simulink model "Simu_SpeedEstimation"  (R2018b)
settings: Solver=FixedStepAuto  StartTime=0.0  StopTime=60  FixedStep=.00005  RelTol=1e-3
undefined symbols (not defined in the file or in its folder): DiscIntNeverNeededParam, sim2mat
libraries: dsparch4 x1, simulink x1
settings Model: Creator=Lubin Kerhuel  LastModifiedBy=Lubin Kerhuel

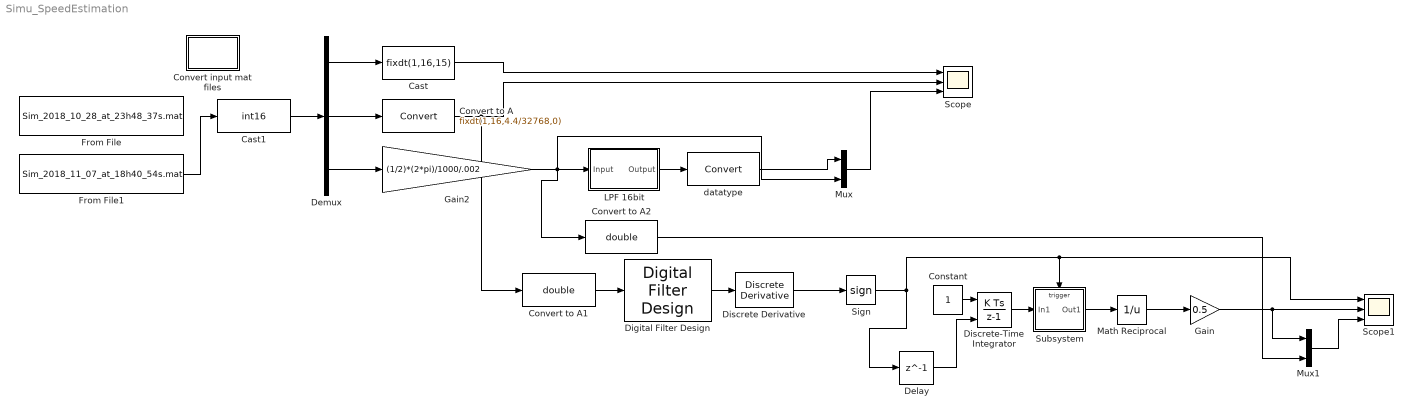
== system Simu_SpeedEstimation ==
  Cast : DataTypeConversion  OutDataTypeStr=fixdt(1,16,15)  ConvertRealWorld=Stored Integer (SI)
  Cast1 : DataTypeConversion  OutDataTypeStr=int16
  Constant : Constant
  Convert input mat files : Subsystem  LoadFcn=sim2mat();
      settings: OpenFcn=sim2mat();
  Convert to A : DataTypeConversion  OutDataTypeStr=fixdt(1,16,4.4/32768,0)  ConvertRealWorld=Stored Integer (SI)
  Convert to A1 : DataTypeConversion  OutDataTypeStr=double
  Convert to A2 : DataTypeConversion  OutDataTypeStr=double
  Delay : Delay  DelayLength=1  InitialCondition=0
  Demux : Demux  Outputs=3
  Digital Filter Design : dsparch4/Digital Filter Design  mwdsp_browser_bugfix_var=off
  Discrete Derivative : simulink/Discrete/Discrete Derivative  gainval=1  ICPrevScaledInput=0  OutMin=[]  OutMax=[]  OutDataType=fixdt(1, 16)  OutScaling=2^-10  DoSatur=off
  Discrete-Time Integrator : DiscreteIntegrator  ExternalReset=rising  SampleTime=-1  ICPrevOutput=DiscIntNeverNeededParam  ICPrevScaledInput=DiscIntNeverNeededParam
  From File : FromFile  FileName=Sim_2018_10_28_at_23h48_37s.mat  SampleTime=.00005
  From File1 : FromFile  FileName=Sim_2018_11_07_at_18h40_54s.mat  SampleTime=.00005
  Gain : Gain  Gain=0.5
  Gain2 : Gain  Gain=(1/2)*(2*pi)/1000/.002  OutDataTypeStr=fixdt(1,16,5)  LockScale=on
  "LPF 16bit " : Subsystem  Tag=FilterWizardSubSystem
      settings: ErrorFcn=dspFilterRealizedInBasicElemsAlgLoopErrFcnCallback
  Math Reciprocal : Math  Operator=reciprocal  SaturateOnIntegerOverflow=on
  Mux : Mux  Inputs=2
  Mux1 : Mux  Inputs=2
  Scope : Scope  NumInputPorts=3
  Scope1 : Scope  NumInputPorts=3
  Sign : Signum
  Subsystem : Subsystem
  datatype : DataTypeConversion
  wires:
  From File1/1 -> Cast1/1
  Demux/1 -> Cast/1
  Demux/2 -> Convert to A/1
  Demux/3 -> Gain2/1
  Cast/1 -> Scope/1
  Convert to A/1 -> Convert to A1/1, Scope/2
  Gain2/1 -> Convert to A2/1, Mux/2, "LPF 16bit "/1(Input)
  Cast1/1 -> Demux/1
  "LPF 16bit "/1(Output) -> datatype/1
  Mux/1 -> Scope/3
  datatype/1 -> Mux/1
  Discrete-Time Integrator/1 -> Subsystem/1(In1)
  Discrete Derivative/1 -> Sign/1
  Constant/1 -> Discrete-Time Integrator/1
  Digital Filter Design/1 -> Discrete Derivative/1
  Convert to A1/1 -> Digital Filter Design/1
  Subsystem/1(Out1) -> Math Reciprocal/1
  Sign/1 -> Delay/1, Subsystem/Trigger, Scope1/1
  Delay/1 -> Discrete-Time Integrator/2
  Math Reciprocal/1 -> Gain/1
  Gain/1 -> Mux1/1, Scope1/2
  Mux1/1 -> Scope1/3
  Convert to A2/1 -> Mux1/2

== system Simu_SpeedEstimation/Convert input mat files ==

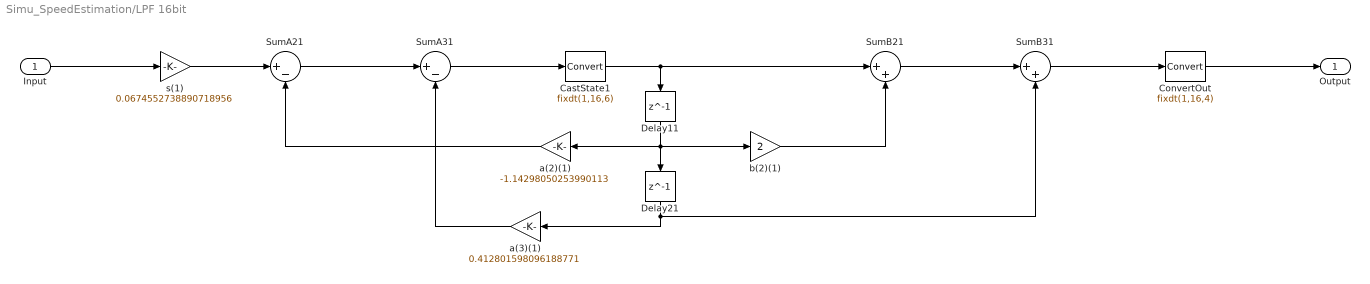
== system Simu_SpeedEstimation/LPF 16bit  ==
  Input : Inport
  CastState1 : DataTypeConversion  OutDataTypeStr=fixdt(1,16,6)
  ConvertOut : DataTypeConversion  OutDataTypeStr=fixdt(1,16,4)
  Delay11 : Delay  DelayLength=1  InitialCondition=0
  Delay21 : Delay  DelayLength=1  InitialCondition=0
  SumA21 : Sum  Inputs=|+-  AccumDataTypeStr=fixdt(1,16,6)  OutDataTypeStr=fixdt(1,16,6)
  SumA31 : Sum  Inputs=|+-  AccumDataTypeStr=fixdt(1,16,6)  OutDataTypeStr=fixdt(1,16,6)
  SumB21 : Sum  Inputs=|++  AccumDataTypeStr=fixdt(1,16,5)  OutDataTypeStr=fixdt(1,16,5)
  SumB31 : Sum  Inputs=|++  AccumDataTypeStr=fixdt(1,16,4)  OutDataTypeStr=fixdt(1,16,4)
  a(2)(1) : Gain  Gain=-1.14298050253990113  ParamDataTypeStr=fixdt(1,16,14)  OutDataTypeStr=fixdt(1,16,6)
  a(3)(1) : Gain  Gain=0.412801598096188771  ParamDataTypeStr=fixdt(0,16,17)  OutDataTypeStr=fixdt(1,16,8)
  b(2)(1) : Gain  Gain=2  ParamDataTypeStr=fixdt(0,16,14)  OutDataTypeStr=fixdt(1,16,5)
  s(1) : Gain  Gain=0.0674552738890718956  ParamDataTypeStr=fixdt(0,16,19)  OutDataTypeStr=fixdt(1,16,8)
  Output : Outport
  wires:
  s(1)/1 -> SumA21/1
  SumA21/1 -> SumA31/1
  SumA31/1 -> CastState1/1
  CastState1/1 -> SumB21/1, Delay11/1
  SumB21/1 -> SumB31/1
  SumB31/1 -> ConvertOut/1
  a(2)(1)/1 -> SumA21/2
  Delay11/1 -> a(2)(1)/1, b(2)(1)/1, Delay21/1
  b(2)(1)/1 -> SumB21/2
  a(3)(1)/1 -> SumA31/2
  Delay21/1 -> a(3)(1)/1, SumB31/2
  ConvertOut/1 -> Output/1
  Input/1 -> s(1)/1

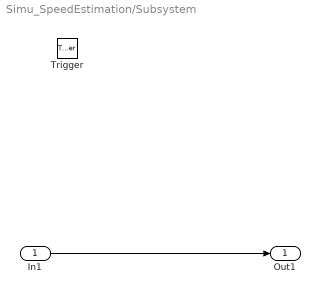
== system Simu_SpeedEstimation/Subsystem ==
  In1 : Inport
  Trigger : TriggerPort  VariantControl=Variant  PortDimensions=1
  Out1 : Outport
  wires:
  In1/1 -> Out1/1
